simulink model "MOD_Hop"  (R2016b)
settings: Solver=ode45  StartTime=0.0  StopTime=60  MaxStep=ts_max  RelTol=1e-8  AbsTol=1e-8  EnableMultiTasking=on
values from neighbouring files (symbols this model uses):
  alpha0 = 90*pi/180    (= 1.57079632679)    [INIT_smm.m]    (also in SIM_Hop.m)
  c = 0.05    [INIT_smm.m]    (also in SIM_Hop.m)
  d = 0.04    [INIT_smm.m]    (also in SIM_Hop.m)
  Delay = 0.015    [INIT_smm.m]    (also in SIM_Hop.m)
  e_ref = 0.04    [SIM_Hop.m]    (also in SIM_smm.m = 0.03)
  Fmaxiso = 22000    [INIT_smm.m]    (also in SIM_Hop.m)
  G = 1    [SIM_Hop.m]    (also in SIM_smm.m)
  g = 9.81    [INIT_smm.m]    (also in PLOT_smm.m; SIM_Hop.m)
  G_F = 1.4    [INIT_smm.m]    (also in SIM_Hop.m; SIM_smm.m = 2.6)
  G_L = 65.1    [INIT_smm.m]    (also in SIM_Hop.m; SIM_smm.m = 130)
  G_V = 2.1    [INIT_smm.m]    (also in SIM_Hop.m; SIM_smm.m = 2.9)
  K = 5    [INIT_smm.m]    (also in SIM_Hop.m)
  l_f = 0.99    [INIT_smm.m]    (also in SIM_Hop.m)
  L_off = 0.075    [INIT_smm.m]    (also in SIM_Hop.m; SIM_smm.m = 0.08)
  l_ref = 0.5    [INIT_smm.m]    (also in SIM_Hop.m)
  l_see_slack = 0.4    [INIT_smm.m]    (also in SIM_Hop.m)
  l_seg = 0.5    [INIT_smm.m]    (also in SIM_Hop.m)
  lambda_F = 1    [SIM_Hop.m]    (also in SIM_smm.m = lambda_Force(i,j))
  lambda_L = 0    [SIM_Hop.m]    (also in SIM_smm.m = lambda_Length(i,j))
  lambda_V = 0    [SIM_Hop.m]    (also in SIM_smm.m = lambda_Velocity(i,j))
  lopt = 0.1    [INIT_smm.m]    (also in SIM_Hop.m)
  m = 80    [INIT_smm.m]    (also in PLOT_smm.m; SIM_Hop.m)
  N = 1.5    [INIT_smm.m]    (also in SIM_Hop.m)
  phi_ref = 110*pi/180    (= 1.91986217719)    [INIT_smm.m]    (also in SIM_Hop.m)
  PreStim = 0.01    [SIM_Hop.m]    (also in SIM_smm.m)
  tau = 0.01    [INIT_smm.m]    (also in SIM_Hop.m)
  V_off = -1.03    [INIT_smm.m]    (also in SIM_Hop.m; SIM_smm.m = -0.6)
  vmax = 12    [INIT_smm.m]    (also in SIM_Hop.m)
  vx0 = 0    [INIT_smm.m]    (also in SIM_Hop.m)
  vy0 = 0    [INIT_smm.m]    (also in SIM_Hop.m)
  w = 0.4    [INIT_smm.m]    (also in SIM_Hop.m)
  y0 = 1.05    [INIT_smm.m]    (also in SIM_Hop.m)
libraries: simulink x4, simulink_extras x2
settings Model: Creator=LL  LastModifiedBy=LL
settings DataIOCC: SaveOutput=off  VisualizeSimOutput=off  TimeSaveName=SIM_time
settings OptimizationCC: LifeSpan=inf
settings DebuggingCC: SaveWithParameterizedLinksMsg=none  UnderspecifiedInitializationDetection=Classic  MergeDetectMultiDrivingBlocksExec=none  SignalResolutionControl=TryResolveAllWithWarning  SolverPrmCheckMsg=warning  MultiTaskDSMMsg=warning  FcnCallInpInsideContextMsg=warning  AssertControl=EnableAll  AllowSymbolicDim=off  StateNameClashWarn=warning  SFUnexpectedBacktrackingDiag=warning  SFNoUnconditionalDefaultTransitionDiag=warning  SFExecutionAtInitializationDiag=none
settings ModelReferenceCC: PropagateSignalLabelsOutOfModel=off
settings GRTTargetCC: TargetLangStandard=C89/C90 (ANSI)
settings ConfigComp: CovMetricSettings=dw  CovHtmlReporting=on  CovSaveCumulativeToWorkspaceVar=on  CovSaveSingleToWorkspaceVar=on  CovExternalEMLEnable=off

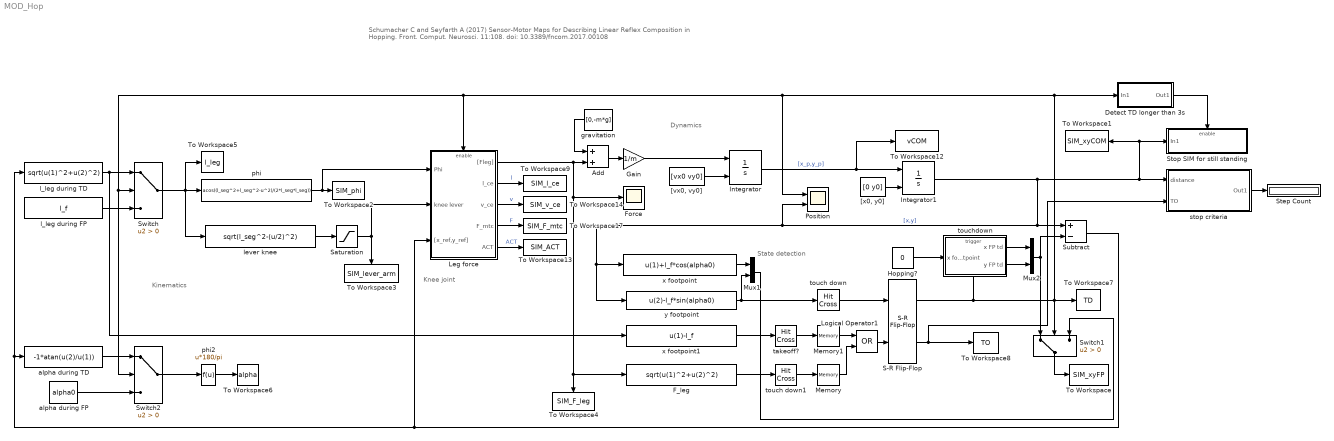
== system MOD_Hop ==
  note: Schumacher C and Seyfarth A (2017) Sensor-Motor Maps for Describing Linear Reflex Composition in Hopping. Front. Comput. Neurosci. 11:108. doi: 10.3389/fncom.2017.00108
  note: Kinematics
  note: State detection
  note: Dynamics
  note: Knee joint
  Add : Sum
  Detect TD longer than 3s : Subsystem
  F_leg : Fcn  Expr=sqrt(u(1)^2+u(2)^2)
  Force : Scope
  Gain : Gain  Gain=1/m
  Hopping? : Constant  Value=0
  Integrator : Integrator  InitialConditionSource=external
  Integrator1 : Integrator  InitialConditionSource=external
  Leg force : Subsystem
  Logical Operator1 : Logic  Operator=OR  AllPortsSameDT=off  OutDataTypeStr=boolean
  Memory : Memory  InheritSampleTime=on
  Memory1 : Memory  X0=-1  InheritSampleTime=on
  Mux1 : Mux  Inputs=2
  Mux2 : Mux  Inputs=2
  Position : Scope  NumInputPorts=2
  S-R Flip-Flop : simulink_extras/Flip Flops/S-R Flip-Flop  initial_condition=0
  Saturation : Saturate  UpperLimit=inf  LowerLimit=0.001
  Step Count : Display
  Stop SIM for still standing : Subsystem
  Subtract : Sum  Inputs=+-
  Switch : Switch  Criteria=u2 > Threshold
  Switch1 : Switch  Criteria=u2 > Threshold
  Switch2 : Switch  Criteria=u2 > Threshold
  To Workspace : ToWorkspace  VariableName=SIM_xyFP  SampleTime=-1
  To Workspace1 : ToWorkspace  VariableName=SIM_xyCOM  SampleTime=-1
      settings: Save2DSignal=2-D array (concatenate along first dimension)
  To Workspace12 : ToWorkspace  VariableName=vCOM  SampleTime=-1
  To Workspace13 : ToWorkspace  VariableName=SIM_ACT  SampleTime=-1
  To Workspace14 : ToWorkspace  VariableName=SIM_v_ce  SampleTime=-1
  To Workspace17 : ToWorkspace  VariableName=SIM_F_mtc  SampleTime=-1
  To Workspace2 : ToWorkspace  VariableName=SIM_phi  SampleTime=-1
  To Workspace3 : ToWorkspace  VariableName=SIM_lever_arm  SampleTime=-1
  To Workspace4 : ToWorkspace  VariableName=SIM_F_leg  SampleTime=-1
  To Workspace5 : ToWorkspace  VariableName=l_leg  SampleTime=-1
  To Workspace6 : ToWorkspace  VariableName=alpha  SampleTime=-1
  To Workspace7 : ToWorkspace  VariableName=TD  SampleTime=-1
  To Workspace8 : ToWorkspace  VariableName=TO  SampleTime=-1
  To Workspace9 : ToWorkspace  VariableName=SIM_l_ce  SampleTime=-1
  "[vx0, vy0]" : Constant  Value=[vx0 vy0]
  "[x0, y0]" : Constant  Value=[0 y0]
  alpha during FP : Constant  Value=alpha0
  alpha during TD : Fcn  Expr=-1*atan(u(2)/u(1))
  gravitation : Constant  Value=[0,-m*g]
  l_leg during FP : Constant  Value=l_f
  l_leg during TD : Fcn  Expr=sqrt(u(1)^2+u(2)^2)
  lever knee : Fcn  Expr=sqrt(l_seg^2-(u/2)^2)
  phi : Fcn  Expr=acos((l_seg^2+l_seg^2-u^2)/(2*l_seg*l_seg))
  phi2 : Fcn  Expr=u*180/pi
  stop criteria : Subsystem
  takeoff? : HitCross  HitCrossingOffset=1e-20  HitCrossingDirection=rising
  touch down : HitCross  HitCrossingDirection=falling
  touch down1 : HitCross  HitCrossingOffset=1e-20  HitCrossingDirection=falling
  touchdown : Subsystem  TreatAsAtomicUnit=on
  x footpoint : Fcn  Expr=u(1)+l_f*cos(alpha0)
  x footpoint1 : Fcn  Expr=u(1)-l_f
  y footpoint : Fcn  Expr=u(2)-l_f*sin(alpha0)
  wires:
  Integrator/1 -> To Workspace12/1, Integrator1/1  "[x_p,y_p]"
  Integrator1/1 -> To Workspace1/1, Stop SIM for still standing/1(In1), stop criteria/1(" distance"), Position/2, y footpoint/1, x footpoint/1, Subtract/1  "[x,y]"
  y footpoint/1 -> touch down/1, Mux1/2
  touch down/1 -> S-R Flip-Flop/1
  x footpoint/1 -> Mux1/1
  touchdown/1(x FP td) -> Mux2/1
  touchdown/2(y FP td) -> Mux2/2
  Mux2/1 -> Switch1/1, Subtract/2
  gravitation/1 -> Add/1
  S-R Flip-Flop/2 -> stop criteria/2(TO), To Workspace8/1
  Add/1 -> Gain/1
  "[vx0, vy0]"/1 -> Integrator/2
  "[x0, y0]"/1 -> Integrator1/2
  Gain/1 -> Integrator/1
  l_leg during FP/1 -> Switch/3
  Saturation/1 -> To Workspace3/1, Leg force/2(knee lever)
  phi/1 -> To Workspace2/1, Leg force/1(Phi)
  lever knee/1 -> Saturation/1
  l_leg during TD/1 -> x footpoint1/1, Switch/1
  Switch/1 -> lever knee/1, To Workspace5/1, phi/1
  Switch1/1 -> To Workspace/1
  Mux1/1 -> Switch1/3
  x footpoint1/1 -> takeoff?/1
  Subtract/1 -> l_leg during TD/1, alpha during TD/1, Leg force/3("[x_ref,y_ref]")
  alpha during TD/1 -> Switch2/1
  phi2/1 -> To Workspace6/1
  alpha during FP/1 -> Switch2/3
  Switch2/1 -> phi2/1
  stop criteria/1(Out1) -> Step Count/1
  Hopping?/1 -> touchdown/1(x footpoint)
  S-R Flip-Flop/1 -> Detect TD longer than 3s/1(In1), Position/1, Switch2/2, Switch/2, Leg force/Enable, To Workspace7/1, Switch1/2, touchdown/Trigger
  F_leg/1 -> touch down1/1
  takeoff?/1 -> Memory1/1
  Logical Operator1/1 -> S-R Flip-Flop/2
  touch down1/1 -> Memory/1
  Memory/1 -> Logical Operator1/2
  Memory1/1 -> Logical Operator1/1
  Detect TD longer than 3s/1(Out1) -> Stop SIM for still standing/Enable
  Leg force/1("[Fleg]") -> To Workspace4/1, F_leg/1, Force/1, Add/2
  Leg force/3(v_ce) -> To Workspace14/1  "v"
  Leg force/2(l_ce) -> To Workspace9/1  "l"
  Leg force/4(F_mtc) -> To Workspace17/1  "F"
  Leg force/5(ACT) -> To Workspace13/1  "ACT"

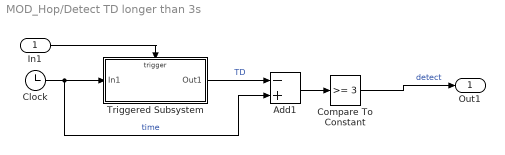
== system MOD_Hop/Detect TD longer than 3s ==
  In1 : Inport
  Add1 : Sum  Inputs=-+
  Clock : Clock
  Compare To Constant : simulink/Logic and Bit Operations/Compare To Constant  relop=>=  const=3  OutDataTypeStr=boolean
  Triggered Subsystem : Subsystem  TreatAsAtomicUnit=on
  Out1 : Outport
  wires:
  Compare To Constant/1 -> Out1/1  "detect"
  Add1/1 -> Compare To Constant/1
  Clock/1 -> Add1/2, Triggered Subsystem/1(In1)  "time"
  In1/1 -> Triggered Subsystem/Trigger
  Triggered Subsystem/1(Out1) -> Add1/1  "TD"

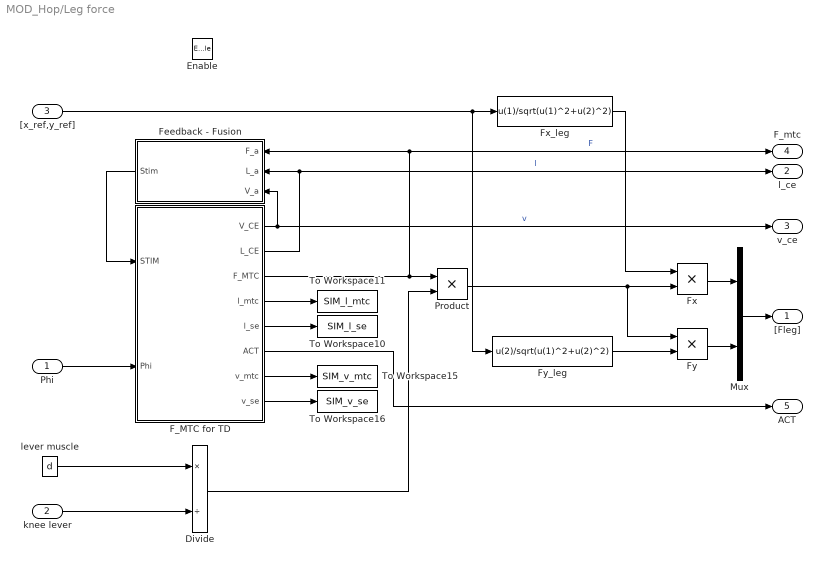
== system MOD_Hop/Leg force ==
  Phi : Inport
  knee lever : Inport  Port=2
  "[x_ref,y_ref]" : Inport  Port=3
  Enable : EnablePort  StatesWhenEnabling=reset  PropagateVarSize=During execution
  Divide : Product  Inputs=*/
  F_MTC for TD : Subsystem  TreatAsAtomicUnit=on
  Feedback - Fusion : Subsystem
  Fx : Product
  Fx_leg : Fcn  Expr=u(1)/sqrt(u(1)^2+u(2)^2)
  Fy : Product
  Fy_leg : Fcn  Expr=u(2)/sqrt(u(1)^2+u(2)^2)
  Mux : Mux  Inputs=2
  Product : Product
  To Workspace10 : ToWorkspace  VariableName=SIM_l_se  SampleTime=-1
  To Workspace11 : ToWorkspace  VariableName=SIM_l_mtc  SampleTime=-1
  To Workspace15 : ToWorkspace  VariableName=SIM_v_mtc  SampleTime=-1
  To Workspace16 : ToWorkspace  VariableName=SIM_v_se  SampleTime=-1
  lever muscle : Constant  Value=d
  "[Fleg]" : Outport  OutputWhenDisabled=reset  InitialOutput=[0 0]
  l_ce : Outport  Port=2
  v_ce : Outport  Port=3
  F_mtc : Outport  Port=4
  ACT : Outport  Port=5
  wires:
  F_MTC for TD/3(F_MTC) -> Product/1, F_mtc/1, Feedback - Fusion/1(F_a)  "F"
  Divide/1 -> Product/2
  lever muscle/1 -> Divide/1
  Mux/1 -> "[Fleg]"/1
  Fx/1 -> Mux/1
  Fx_leg/1 -> Fx/1
  Product/1 -> Fy/1, Fx/2
  Fy/1 -> Mux/2
  Fy_leg/1 -> Fy/2
  knee lever/1 -> Divide/2
  Phi/1 -> F_MTC for TD/2(Phi)
  "[x_ref,y_ref]"/1 -> Fy_leg/1, Fx_leg/1
  Feedback - Fusion/1(Stim) -> F_MTC for TD/1(STIM)
  F_MTC for TD/4(l_mtc) -> To Workspace11/1
  F_MTC for TD/5(l_se) -> To Workspace10/1
  F_MTC for TD/6(ACT) -> ACT/1
  F_MTC for TD/1(V_CE) -> v_ce/1, Feedback - Fusion/3(V_a)  "v"
  F_MTC for TD/2(L_CE) -> l_ce/1, Feedback - Fusion/2(L_a)  "l"
  F_MTC for TD/7(v_mtc) -> To Workspace15/1
  F_MTC for TD/8(v_se) -> To Workspace16/1

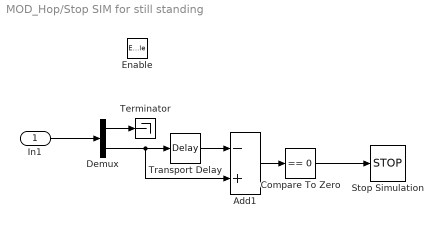
== system MOD_Hop/Stop SIM for still standing ==
  In1 : Inport
  Enable : EnablePort
  Add1 : Sum  Inputs=-+
  Compare To Zero : simulink/Logic and Bit Operations/Compare To Zero  relop===  OutDataTypeStr=boolean
  Demux : Demux  Outputs=2
  Stop Simulation : Stop
  Terminator : Terminator
  Transport Delay : TransportDelay  TransDelayFeedthrough=on
  wires:
  Compare To Zero/1 -> Stop Simulation/1
  In1/1 -> Demux/1
  Demux/1 -> Terminator/1
  Demux/2 -> Transport Delay/1, Add1/2
  Add1/1 -> Compare To Zero/1
  Transport Delay/1 -> Add1/1

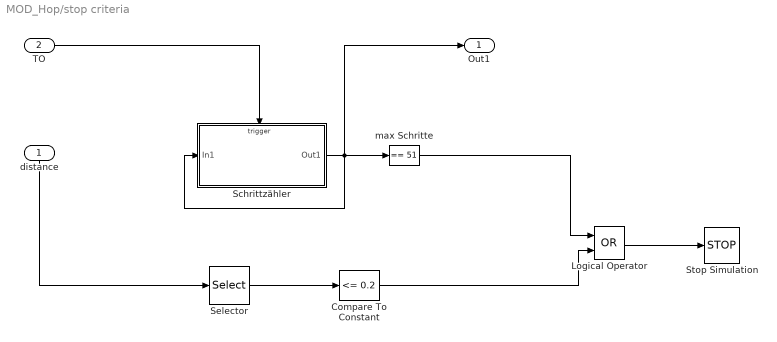
== system MOD_Hop/stop criteria ==
  " distance" : Inport
  TO : Inport  Port=2
  Compare To Constant : simulink/Logic and Bit Operations/Compare To Constant  relop=<=  const=0.2  OutDataTypeStr=boolean
  Logical Operator : Logic  Operator=OR  AllPortsSameDT=off  OutDataTypeStr=boolean
  Schrittzähler : Subsystem  TreatAsAtomicUnit=on
  Selector : Selector  InputPortWidth=2  IndexOptions=Index vector (dialog)  Indices=[2]  OutputSizes=1
  Stop Simulation : Stop
  max Schritte : simulink/Logic and Bit Operations/Compare To Constant  relop===  const=51  OutDataTypeStr=uint8
  Out1 : Outport
  wires:
  Schrittzähler/1(Out1) -> Out1/1, max Schritte/1, Schrittzähler/1(In1)
  Selector/1 -> Compare To Constant/1
  max Schritte/1 -> Logical Operator/1
  Compare To Constant/1 -> Logical Operator/2
  Logical Operator/1 -> Stop Simulation/1
  " distance"/1 -> Selector/1
  TO/1 -> Schrittzähler/Trigger

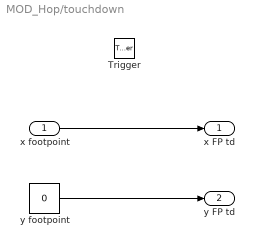
== system MOD_Hop/touchdown ==
  x footpoint : Inport
  Trigger : TriggerPort  VariantControl=Variant
  y footpoint : Constant  Value=0
  x FP td : Outport
  y FP td : Outport  Port=2  InitialOutput=[0]
  wires:
  x footpoint/1 -> x FP td/1
  y footpoint/1 -> y FP td/1

== system MOD_Hop/Detect TD longer than 3s/Triggered Subsystem ==
  In1 : Inport
  Trigger : TriggerPort  VariantControl=Variant
  Out1 : Outport  InitialOutput=[0]
  wires:
  In1/1 -> Out1/1

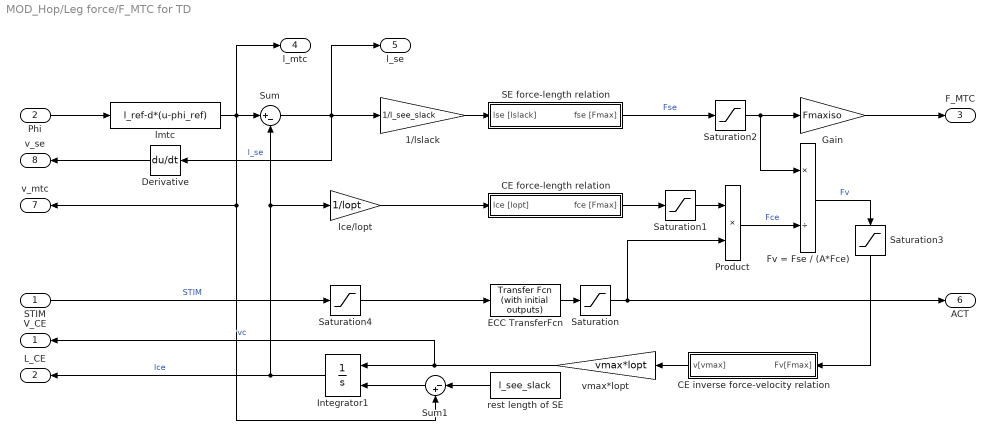
== system MOD_Hop/Leg force/F_MTC for TD ==
  STIM : Inport
  Phi : Inport  Port=2
  1/lslack : Gain  Gain=1/l_see_slack  SaturateOnIntegerOverflow=on  OutDataTypeStr=Inherit: Same as input  ParamDataTypeStr=Inherit: Same as input
  CE force-length relation : Subsystem
  CE inverse force-velocity relation : Subsystem
  Derivative : Derivative
  ECC TransferFcn : simulink_extras/Additional Linear/Transfer Fcn (with initial outputs)  N=[1]  D="[tau  1]"  Y0=0  U0=PreStim
      settings: AttributesFormatString=pre-activation: %<Y0>
  Fv = Fse / (A*Fce) : Product  Inputs=*/  SaturateOnIntegerOverflow=on  InputSameDT=on  OutDataTypeStr=Inherit: Same as first input
  Gain : Gain  Gain=Fmaxiso
  Integrator1 : Integrator  InitialConditionSource=external
  Product : Product
  SE force-length relation : Subsystem
  Saturation : Saturate  UpperLimit=inf  LowerLimit=0.001  ZeroCross=off
  Saturation1 : Saturate  UpperLimit=1  LowerLimit=0  ZeroCross=off
  Saturation2 : Saturate  UpperLimit=N  LowerLimit=0
  Saturation3 : Saturate  UpperLimit=N  LowerLimit=0  ZeroCross=off
  Saturation4 : Saturate  UpperLimit=1  LowerLimit=0  ZeroCross=off
  Sum : Sum  Inputs=|+-
  Sum1 : Sum  Inputs=|-+  SaturateOnIntegerOverflow=on  InputSameDT=on  OutDataTypeStr=Inherit: Same as first input
  lce/lopt : Gain  Gain=1/lopt  SaturateOnIntegerOverflow=on  OutDataTypeStr=Inherit: Same as input  ParamDataTypeStr=Inherit: Same as input
  lmtc : Fcn  Expr=l_ref-d*(u-phi_ref)
  rest length of SE : Constant  Value=l_see_slack
  vmax*lopt : Gain  Gain=vmax*lopt  SaturateOnIntegerOverflow=on  OutDataTypeStr=Inherit: Same as input  ParamDataTypeStr=Inherit: Same as input
  V_CE : Outport  InitialOutput=[-1]
  L_CE : Outport  Port=2  InitialOutput=[-1]
  F_MTC : Outport  Port=3  InitialOutput=[-1]
  l_mtc : Outport  Port=4
  l_se : Outport  Port=5
  ACT : Outport  Port=6  InitialOutput=[-1]
  v_mtc : Outport  Port=7
  v_se : Outport  Port=8
  wires:
  lce/lopt/1 -> CE force-length relation/1(lce [lopt])
  1/lslack/1 -> SE force-length relation/1(lse [lslack])
  Sum/1 -> l_se/1, Derivative/1, 1/lslack/1  "l_se"
  Phi/1 -> lmtc/1
  CE force-length relation/1(fce [Fmax]) -> Saturation1/1
  Fv = Fse / (A*Fce)/1 -> Saturation3/1  "Fv"
  Saturation1/1 -> Product/1
  Gain/1 -> F_MTC/1
  vmax*lopt/1 -> V_CE/1, Integrator1/1  "vc"
  Integrator1/1 -> Sum/2, lce/lopt/1, L_CE/1  "lce"
  rest length of SE/1 -> Sum1/1
  Sum1/1 -> Integrator1/2
  CE inverse force-velocity relation/1(v[vmax]) -> vmax*lopt/1
  ECC TransferFcn/1 -> Saturation/1
  STIM/1 -> Saturation4/1  "STIM"
  Product/1 -> Fv = Fse / (A*Fce)/2  "Fce"
  Saturation2/1 -> Fv = Fse / (A*Fce)/1, Gain/1
  Saturation/1 -> Product/2, ACT/1
  Saturation4/1 -> ECC TransferFcn/1
  Saturation3/1 -> CE inverse force-velocity relation/1(Fv[Fmax])
  lmtc/1 -> l_mtc/1, v_mtc/1, Sum1/2, Sum/1
  SE force-length relation/1(fse [Fmax]) -> Saturation2/1  "Fse"
  Derivative/1 -> v_se/1

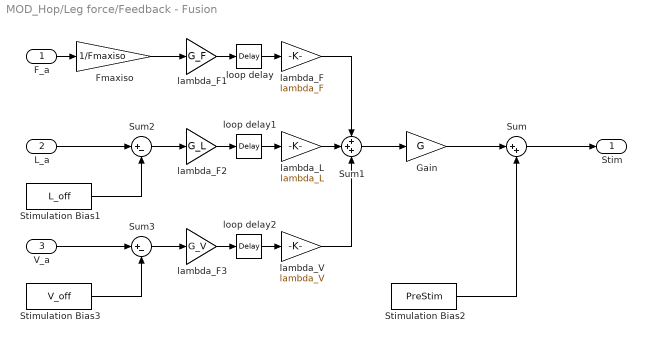
== system MOD_Hop/Leg force/Feedback - Fusion ==
  F_a : Inport
  L_a : Inport  Port=2
  V_a : Inport  Port=3
  Fmaxiso : Gain  Gain=1/Fmaxiso
  Gain : Gain  Gain=G
  Stimulation Bias1 : Constant  Value=L_off
  Stimulation Bias2 : Constant  Value=PreStim
  Stimulation Bias3 : Constant  Value=V_off
  Sum : Sum  Inputs=|++
  Sum1 : Sum  Inputs=+++
  Sum2 : Sum  Inputs=|+-
  Sum3 : Sum  Inputs=|+-
  lambda_F : Gain  Gain=lambda_F
  lambda_F1 : Gain  Gain=G_F
  lambda_F2 : Gain  Gain=G_L
  lambda_F3 : Gain  Gain=G_V
  lambda_L : Gain  Gain=lambda_L
  lambda_V : Gain  Gain=lambda_V
  loop delay : TransportDelay  DelayTime=Delay
  loop delay1 : TransportDelay  DelayTime=Delay
  loop delay2 : TransportDelay  DelayTime=Delay
  Stim : Outport
  wires:
  F_a/1 -> Fmaxiso/1
  loop delay/1 -> lambda_F/1
  Stimulation Bias2/1 -> Sum/2
  lambda_F/1 -> Sum1/1
  Fmaxiso/1 -> lambda_F1/1
  lambda_F1/1 -> loop delay/1
  Sum/1 -> Stim/1
  Gain/1 -> Sum/1
  loop delay1/1 -> lambda_L/1
  loop delay2/1 -> lambda_V/1
  Sum3/1 -> lambda_F3/1
  V_a/1 -> Sum3/1
  L_a/1 -> Sum2/1
  Sum2/1 -> lambda_F2/1
  Stimulation Bias1/1 -> Sum2/2
  Stimulation Bias3/1 -> Sum3/2
  lambda_L/1 -> Sum1/2
  lambda_V/1 -> Sum1/3
  lambda_F2/1 -> loop delay1/1
  lambda_F3/1 -> loop delay2/1
  Sum1/1 -> Gain/1

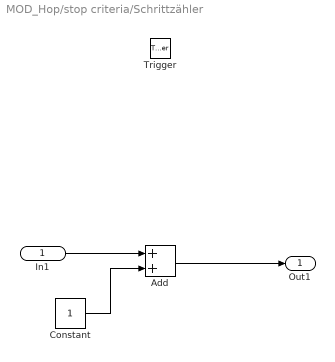
== system MOD_Hop/stop criteria/Schrittzähler ==
  In1 : Inport  LatchByDelayingOutsideSignal=on
  Trigger : TriggerPort  VariantControl=Variant
  Add : Sum
  Constant : Constant
  Out1 : Outport
  wires:
  In1/1 -> Add/1
  Constant/1 -> Add/2
  Add/1 -> Out1/1

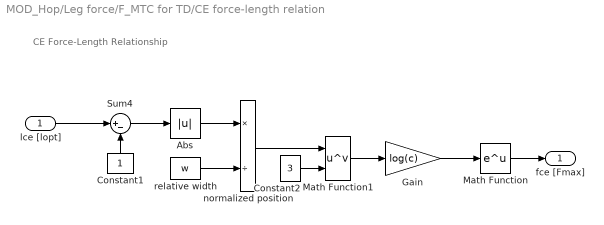
== system MOD_Hop/Leg force/F_MTC for TD/CE force-length relation ==
  note: CE Force-Length Relationship
  lce [lopt] : Inport
  Abs : Abs
  Constant1 : Constant
  Constant2 : Constant  Value=3
  Gain : Gain  Gain=log(c)
  Math Function : Math  SaturateOnIntegerOverflow=on
  Math Function1 : Math  Operator=pow  SaturateOnIntegerOverflow=on
  Sum4 : Sum  Inputs=|+-  SaturateOnIntegerOverflow=on  InputSameDT=on  OutDataTypeStr=Inherit: Same as first input
  normalized position : Product  Inputs=*/
  relative width : Constant  Value=w
  fce [Fmax] : Outport
  wires:
  lce [lopt]/1 -> Sum4/1
  relative width/1 -> normalized position/2
  Constant1/1 -> Sum4/2
  Sum4/1 -> Abs/1
  Abs/1 -> normalized position/1
  normalized position/1 -> Math Function1/1
  Constant2/1 -> Math Function1/2
  Math Function1/1 -> Gain/1
  Gain/1 -> Math Function/1
  Math Function/1 -> fce [Fmax]/1

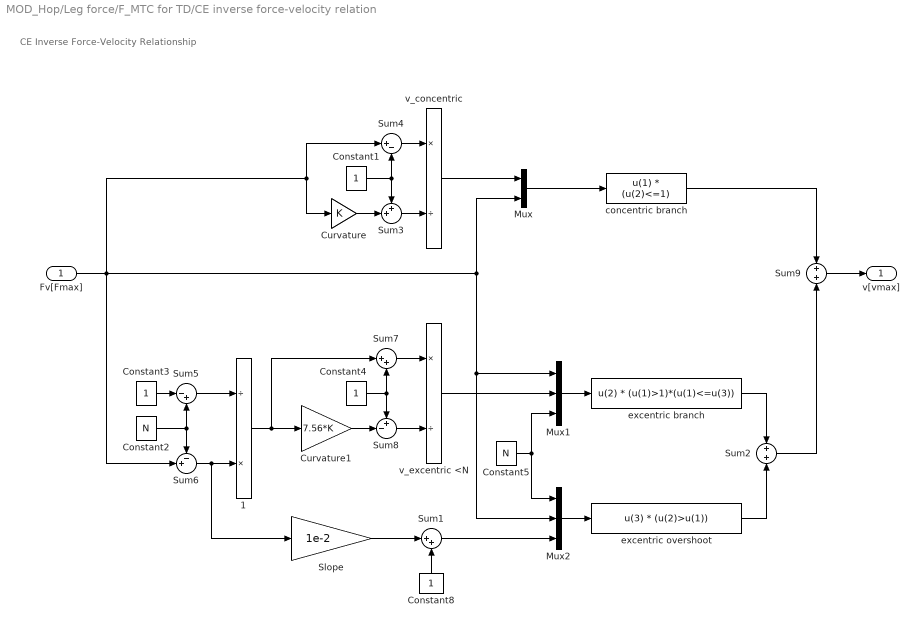
== system MOD_Hop/Leg force/F_MTC for TD/CE inverse force-velocity relation ==
  note: CE Inverse Force-Velocity Relationship
  Fv[Fmax] : Inport
  1 : Product  Inputs=/*
  Constant{1,3..4,8} (4 alike) : Constant
  Constant2 : Constant  Value=N
  Constant5 : Constant  Value=N
  Curvature : Gain  Gain=K  SaturateOnIntegerOverflow=on  OutDataTypeStr=Inherit: Same as input  ParamDataTypeStr=Inherit: Same as input
  Curvature1 : Gain  Gain=7.56*K  SaturateOnIntegerOverflow=on  OutDataTypeStr=Inherit: Same as input  ParamDataTypeStr=Inherit: Same as input
  Mux : Mux  Inputs=2
  Mux1 : Mux  Inputs=3
  Mux2 : Mux  Inputs=3
  Slope : Gain  Gain=1e-2  SaturateOnIntegerOverflow=on  OutDataTypeStr=Inherit: Same as input  ParamDataTypeStr=Inherit: Same as input
  Sum1 : Sum  Inputs=|++  SaturateOnIntegerOverflow=on  InputSameDT=on  OutDataTypeStr=Inherit: Same as first input
  Sum2 : Sum  SaturateOnIntegerOverflow=on  InputSameDT=on  OutDataTypeStr=Inherit: Same as first input
  Sum3 : Sum  Inputs=++|  SaturateOnIntegerOverflow=on  InputSameDT=on  OutDataTypeStr=Inherit: Same as first input
  Sum4 : Sum  Inputs=|+-  SaturateOnIntegerOverflow=on  InputSameDT=on  OutDataTypeStr=Inherit: Same as first input
  Sum5 : Sum  Inputs=|-+  SaturateOnIntegerOverflow=on  InputSameDT=on  OutDataTypeStr=Inherit: Same as first input
  Sum6 : Sum  Inputs=-+|  SaturateOnIntegerOverflow=on  InputSameDT=on  OutDataTypeStr=Inherit: Same as first input
  Sum7 : Sum  Inputs=|++  SaturateOnIntegerOverflow=on  InputSameDT=on  OutDataTypeStr=Inherit: Same as first input
  Sum8 : Sum  Inputs=+-|  SaturateOnIntegerOverflow=on  InputSameDT=on  OutDataTypeStr=Inherit: Same as first input
  Sum9 : Sum  SaturateOnIntegerOverflow=on  InputSameDT=on  OutDataTypeStr=Inherit: Same as first input
  concentric branch : Fcn  Expr=u(1) * (u(2)<=1)
  excentric branch : Fcn  Expr=u(2) * (u(1)>1)*(u(1)<=u(3))
  excentric overshoot : Fcn  Expr=u(3) * (u(2)>u(1))
  v_concentric : Product  Inputs=*/
  v_excentric <N : Product  Inputs=*/
  v[vmax] : Outport
  wires:
  Curvature/1 -> Sum3/2
  Constant1/1 -> Sum4/2, Sum3/1
  Sum4/1 -> v_concentric/1
  Sum3/1 -> v_concentric/2
  1/1 -> Sum7/1, Curvature1/1
  Constant4/1 -> Sum7/2, Sum8/1
  Curvature1/1 -> Sum8/2
  Sum8/1 -> v_excentric <N/2
  Sum7/1 -> v_excentric <N/1
  v_concentric/1 -> Mux/1
  Fv[Fmax]/1 -> Sum4/1, Curvature/1, Sum6/2, Mux/2, Mux1/1, Mux2/2
  Sum9/1 -> v[vmax]/1
  Sum2/1 -> Sum9/2
  excentric overshoot/1 -> Sum2/2
  Slope/1 -> Sum1/1
  Constant8/1 -> Sum1/2
  Sum6/1 -> 1/2, Slope/1
  Constant2/1 -> Sum6/1, Sum5/2
  Sum5/1 -> 1/1
  Constant3/1 -> Sum5/1
  Mux/1 -> concentric branch/1
  Mux1/1 -> excentric branch/1
  v_excentric <N/1 -> Mux1/2
  Mux2/1 -> excentric overshoot/1
  concentric branch/1 -> Sum9/1
  excentric branch/1 -> Sum2/1
  Constant5/1 -> Mux1/3, Mux2/1
  Sum1/1 -> Mux2/3

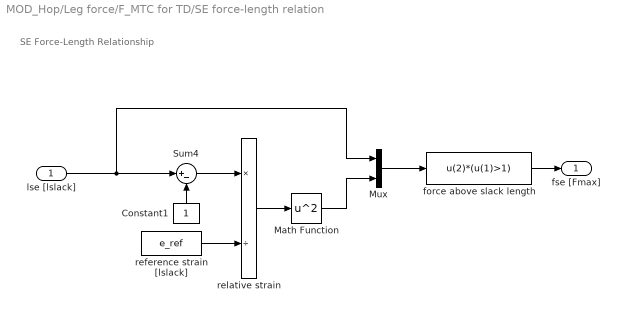
== system MOD_Hop/Leg force/F_MTC for TD/SE force-length relation ==
  note: SE Force-Length Relationship
  lse [lslack] : Inport
  Constant1 : Constant
  Math Function : Math  Operator=square  SaturateOnIntegerOverflow=on
  Mux : Mux  Inputs=2
  Sum4 : Sum  Inputs=|+-  SaturateOnIntegerOverflow=on  InputSameDT=on  OutDataTypeStr=Inherit: Same as first input
  force above slack length : Fcn  Expr=u(2)*(u(1)>1)
  reference strain [lslack] : Constant  Value=e_ref
  relative strain : Product  Inputs=*/
  fse [Fmax] : Outport
  wires:
  Mux/1 -> force above slack length/1
  Math Function/1 -> Mux/2
  lse [lslack]/1 -> Mux/1, Sum4/1
  relative strain/1 -> Math Function/1
  reference strain [lslack]/1 -> relative strain/2
  Sum4/1 -> relative strain/1
  Constant1/1 -> Sum4/2
  force above slack length/1 -> fse [Fmax]/1
